simulink model "rtwdemo_parentheses"  (Simulink 7.6)
settings: Solver=FixedStepDiscrete  StartTime=0.0  StopTime=0.01  FixedStep=0.01  RelTol=1e-3  SampleTimeConstraint=STIndependent
libraries: rtwdemowidgets x2
Description:
  | Parentheses Control
settings Model: Creator=The MathWorks Inc.  ExtModeAutoUpdateStatusClock=off
settings DataIOCC: SaveOutput=off  SaveTime=off
settings OptimizationCC: InlineParams=on  InlineInvariantSignals=on  PassReuseOutputArgsAs=Individual arguments  StateBitsets=on  DataBitsets=on  UseTempVars=on  ZeroExternalMemoryAtStartup=off  ZeroInternalMemoryAtStartup=off  NoFixptDivByZeroProtection=on  EfficientFloat2IntCast=on  EfficientMapNaN2IntZero=off  OptimizeModelRefInitCode=on  LifeSpan=1
settings DebuggingCC: SolverPrmCheckMsg=none  StrictBusMsg=ErrorOnBusTreatedAsVector
settings HardwareCC: ProdIntDivRoundTo=Zero  ProdEndianess=LittleEndian  ProdHWDeviceType=Generic->32-bit Embedded Processor  TargetHWDeviceType=Generic->32-bit Embedded Processor
settings SFSimCC: SimParseCustomCode=off
settings RTWCC: SystemTargetFile=ert.tlc  TemplateMakefile=ert_default_tmf  Description=Real-Time Workshop Embedded Coder (no auto configuration)  GenerateReport=on  RTWVerbose=off  ProcessScript=ert_make_rtw_hook  IncludeHyperlinkInReport=on  LaunchReport=on
settings CodeAppCC: ForceParamTrailComments=on  IgnoreCustomStorageClasses=off  IgnoreTestpoints=on  SimulinkDataObjDesc=on  CustomSymbolStrGlobalVar=rt$N$M  CustomSymbolStrType=$N$M  CustomSymbolStrFcn=$N$M$F  CustomSymbolStrMacro=$N$M  InsertBlockDesc=on
settings ERTTargetCC: TargetFcnLib=ansi_tfl_tmw.mat  MultiwordLength=2048  GenerateSampleERTMain=on  IncludeMdlTerminateFcn=off  SupportNonFinite=off  SupportComplex=off  InlinedParameterPlacement=NonHierarchical  ERTCustomFileTemplate=example_file_process.tlc  ConvertIfToSwitch=off

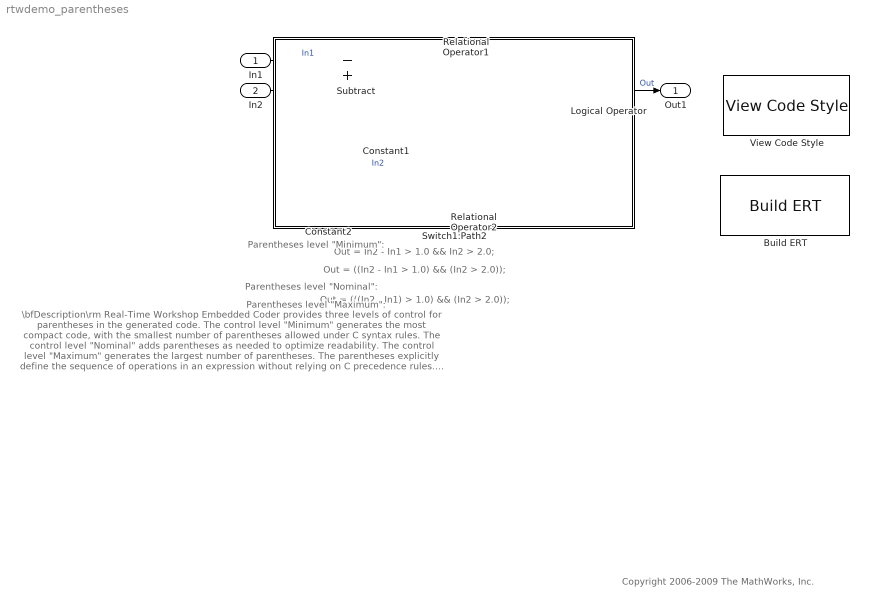
== system rtwdemo_parentheses ==
  note: \bfDescription\rm
      | Real-Time Workshop Embedded Coder provides three levels of control for parentheses in
      | the generated code.  The control level "Minimum" generates the most compact code, with
      | the smallest number of parentheses allowed under C syntax rules.  The control level
      | "Nominal" adds parentheses as needed to optimize readability.  The control level
      | "Maximum" generates the largest number of parentheses.   The parentheses explicitly define
      | the sequence of operations in an expression without relying on C precedence rules.
      | Specifying control level "Maximum" provides full compliance with the MISRA-C(TM) standard.
      |
      | \bfInstructions\rm
      | 1. View and set the parentheses level by double-clicking the yellow button to the right.
      | 2. Generate code by double-clicking the blue button to the right.
      |     An HTML report is displayed automatically.
      | 3. Inspect the generated source files, comparing them with the three code examples above.
  note: Out = In2 - In1 > 1.0 && In2 > 2.0;
  note: Out = ((In2 - In1 > 1.0) && (In2 > 2.0));
  note: Out = (((In2 - In1) > 1.0) && (In2 > 2.0));
  note: Parentheses level "Minimum":
  note: Parentheses level "Nominal":
  note: Parentheses level "Maximum":
  note: Copyright 2006-2009 The MathWorks, Inc.
  In1 : Inport  OutDataTypeStr=double  PortDimensions=1
  In2 : Inport  Port=2  OutDataTypeStr=double  PortDimensions=1
  Build ERT : rtwdemowidgets/Build ERT  SystemSampleTime=-1  attrib_overrides={'ParenthesesLevel'}
  Constant1 : Constant  OutDataTypeStr=double
  Constant2 : Constant  Value=2  OutDataTypeStr=double
  Logical Operator : Logic  AllPortsSameDT=off  OutDataTypeStr=boolean
  Relational Operator1 : RelationalOperator  Operator=>  InputSameDT=on
  Relational Operator2 : RelationalOperator  Operator=>  InputSameDT=on
  Subtract : Sum  Inputs=-+
  Switch1:Path2 : Subsystem
      settings: AttributesFormatString=\n  OpenFcn=disp('');
      mask Display: disp(' ')
  View Code Style : rtwdemowidgets/View Code Style  SystemSampleTime=-1
  Out1 : Outport
  wires:
  In2/1 -> Relational Operator2/1, Subtract/2  "In2"
  Constant2/1 -> Relational Operator2/2
  Logical Operator/1 -> Out1/1  "Out"
  Relational Operator2/1 -> Logical Operator/2
  Relational Operator1/1 -> Logical Operator/1
  Constant1/1 -> Relational Operator1/2
  In1/1 -> Subtract/1  "In1"
  Subtract/1 -> Relational Operator1/1

== system rtwdemo_parentheses/Switch1:Path2 ==
